simulink model "Signalflussplan"  (R2026a)
settings: Solver=VariableStepAuto  StopTime=1.0
values from neighbouring files (symbols this model uses):
  b1 = 2.39e6    (= 2390000)    [variablen2.m]
  c_o = 36.5e6    (= 36500000)    [variablen2.m]
  c_p = 75e6    (= 75000000)    [variablen2.m]
  FN = F_N    (= 63000)    [variablen2.m]
  i_vmax = 1    [variablen2.m]
  K_L = 1    [variablen2.m]
  K_sv = 0.796    [variablen2.m]
  m_g = m_k + m_p    (= 268.7)    [variablen2.m]
settings Model: Creator=johannakruger  LastModifiedBy=johannakruger
settings DataIOCC: ExternalInput=[0 0]  InitialState=[]  LoadExternalInput=on  LoadInitialState=on
settings OptimizationCC: BufferReuse=off
settings DebuggingCC: InitInArrayFormatMsg=none

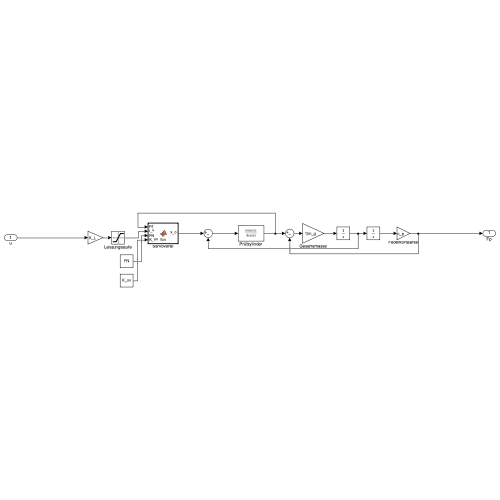
[thumbnail: Simulink's stored preview of the top-level diagram]
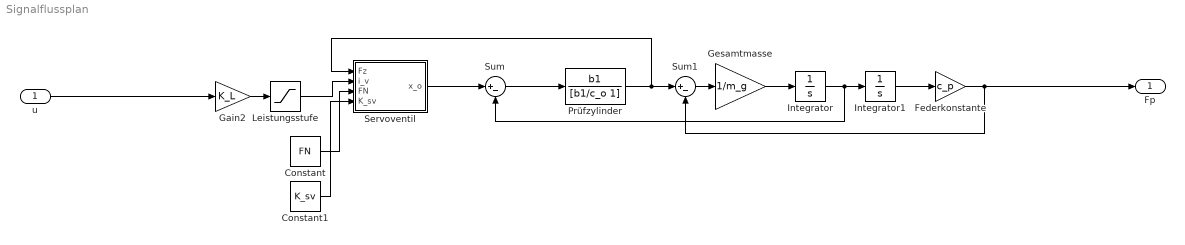
== system Signalflussplan ==
  u : Inport
  Constant : Constant  Value=FN
  Constant1 : Constant  Value=K_sv
  Federkonstante : Gain  Gain=c_p
  Gain2 : Gain  Gain=K_L
  Gesamtmasse : Gain  Gain=1/m_g
  Integrator : Integrator
  Integrator1 : Integrator
  Leistungsstufe : Saturate  UpperLimit=i_vmax  LowerLimit=-i_vmax
  Prüfzylinder : TransferFcn  Numerator=b1  Denominator=[b1/c_o 1]
  Servoventil : MATLAB Function  TreatAsAtomicUnit=on
  Sum : Sum  Inputs=|+-
  Sum1 : Sum  Inputs=|+-
  Fp : Outport
  wires:
  Leistungsstufe/1 -> Servoventil/2(i_v)
  Gesamtmasse/1 -> Integrator/1
  Integrator1/1 -> Federkonstante/1
  Servoventil/1(x_o) -> Sum/1
  Sum/1 -> Prüfzylinder/1
  Integrator/1 -> Sum/2, Integrator1/1
  Sum1/1 -> Gesamtmasse/1
  Federkonstante/1 -> Fp/1, Sum1/2
  Prüfzylinder/1 -> Servoventil/1(Fz), Sum1/1
  Constant/1 -> Servoventil/3(FN)
  Constant1/1 -> Servoventil/4(K_sv)
  Gain2/1 -> Leistungsstufe/1
  u/1 -> Gain2/1

== matlab function Signalflussplan/Servoventil ==
  data: Fz input; i_v input; x_o output; FN input; K_sv input
function x_o = fcn(Fz, i_v, FN, K_sv)

A = 1 - Fz/FN * sign(i_v);

if A <= 0
    x_o = 0;
else
    x_o = i_v * K_sv * sqrt(A);
end
